simulink model "E3_QHW"  (R2025a)
settings: Solver=ode4  StartTime=0.0  StopTime=15  FixedStep=0.002  RelTol=1e-3  EnableMultiTasking=on
undefined symbols (not defined in the file): alpha_meas, g, HIL, Jp_cm, kt, l, mode, mp, mr, nis, p, qc_get_step_size, r, ref, Rm, seq, TET, theta_meas, tmodel, twall, Vm, xhat
libraries: quarc_library x7, simulink x6
settings Model: SimulationMode=external  ExtModeTrigDuration=10000  Creator=sebas  LastModifiedBy=sebas
settings SolverCC: AlgebraicLoopSolver=TrustRegion  PositivePriorityOrder=on
settings DataIOCC: ReturnWorkspaceOutputs=off
settings DebuggingCC: UnconnectedInputMsg=warning  UnconnectedOutputMsg=warning  UnconnectedLineMsg=warning  ArithmeticOperatorsInVariantConditions=warning
settings ModelReferenceCC: EnableRefExpFcnMdlSchedulingChecks=on
settings SFSimCC: SimUseLocalCustomCode=off  CustomCodeUndefinedFunction=UseInterfaceOnly
settings RTWCC: SystemTargetFile=quarc_win64.tlc  TemplateMakefile=quarc_default_tmf  RTWUseLocalCustomCode=off  Toolchain=QUARC win64 | nmake (64-bit Windows)  BuildConfiguration=Faster Runs  GPUComputeCapability=3.5  Description=QUARC Win64 Target Using Toolchain
settings CodeAppCC: StateflowObjectComments=on
settings STFCustomTargetCC: SystemTargetFile=quarc_win64.tlc  TargetLangStandard=C99 (ISO)  MultiwordLength=2048.0  DynamicStringBufferSize=256.0  ConcurrentExecutionCompliant=on  UseToolchainInfoCompliant=on
settings GRTTargetCC: ExtMode=on  ExtModeMexFile=quarc_comm  ParMdlRefBuildCompliant=off  CompOptLevelCompliant=off  CombineOutputUpdateFcns=off  MatFileLogging=off  CPPClassGenCompliant=off  GRTInterface=on
settings ConfigComp: CovMetricSettings=dswe

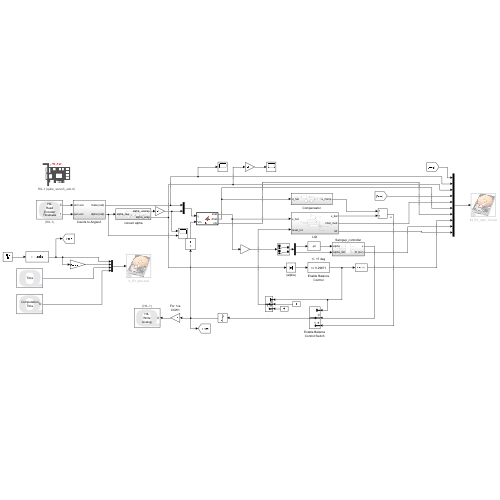
[thumbnail: Simulink's stored preview of the top-level diagram]
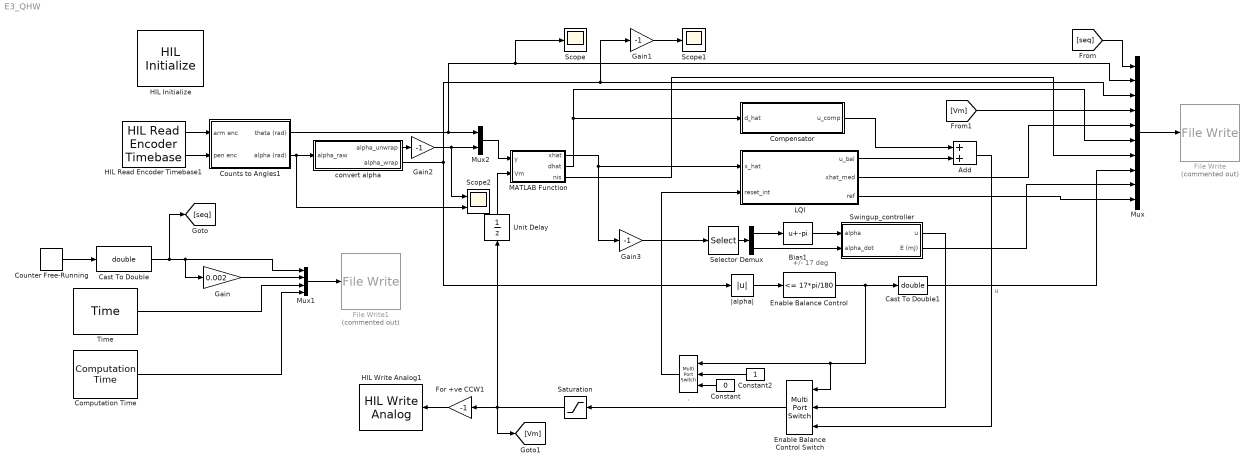
== system E3_QHW ==
  note: +/- 17 deg
  . : MultiPortSwitch  DataPortOrder=Zero-based contiguous  Inputs=2  zeroidx=on  SaturateOnIntegerOverflow=off  InputSameDT=off
  Add : Sum
  Bias1 : Bias  Bias=-pi  SaturateOnIntegerOverflow=off
  Cast To Double : DataTypeConversion  OutDataTypeStr=double  SaturateOnIntegerOverflow=off  RndMeth=Floor
  Cast To Double1 : DataTypeConversion  OutDataTypeStr=double  SaturateOnIntegerOverflow=off  RndMeth=Floor
  Compensator : Subsystem
  Computation Time : quarc_library/Sources/Time/Computation Time  sample_time=qc_get_step_size  use_model=on  use_cpu_time=off
  Constant : Constant  Value=0
  Constant2 : Constant
  Counter Free-Running : simulink/Sources/Counter Free-Running  NumBits=16  tsamp=0.002
  Counts to Angles1 : Subsystem
  Demux : Demux  Outputs=2
  Enable Balance Control : simulink/Logic and Bit Operations/Compare To Constant  relop=<=  const=17*pi/180  OutDataTypeStr=boolean  ZeroCross=off
  Enable Balance Control Switch : MultiPortSwitch  DataPortOrder=Zero-based contiguous  Inputs=2  zeroidx=on  SaturateOnIntegerOverflow=off  InputSameDT=off
  File Write : quarc_library/Sinks/To Target/File Write  Commented=on  source=Specify via dialog (do not evaluate)  file_name=fid_E3_qhw_10.mat  variable_name=seq,theta_meas,alpha_meas,Vm,xhat.dhat,nis,mode,E,ref  decimation=1  sample_time=0.002  file_format=MAT-file v.4  options=No header or footer  append=off  encoding=Default  bitrate=0
      settings: AttributesFormatString=%<file_name>  SourceProductName=QUARC Targets
  File Write1 : quarc_library/Sinks/To Target/File Write  Commented=on  source=Specify via dialog (do not evaluate)  file_name=rt_E3_qhw.mat  variable_name=seq,tmodel,twall,TET  decimation=1  sample_time=0.002  file_format=MAT-file v.4  options=No header or footer  append=off  encoding=Default  bitrate=0
      settings: AttributesFormatString=%<file_name>  SourceProductName=QUARC Targets
  For +ve CCW1 : Gain  Gain=-1
  Gain : Gain  Gain=0.002
  Gain1 : Gain  Gain=-1
  Gain2 : Gain  Gain=-1
  Gain3 : Gain  Gain=-1
  HIL Initialize : quarc_library/Data Acquisition/Generic/Configuration/HIL Initialize  object_name=HIL-1  board_type=qube_servo3_usb  board_number=0  board_options=deadband_compensation=0.3;pwm_en=0;enc0_velocity=3.0;enc1_velocity=3.0;min_diode_compensation=0.3;max_diode_compensation=1.5  exclusive=off  active=on  hardware_clocks=[0]  clock_modes=[]  initial_clock_frequencies=[]  set_clock_params_at_start=off  set_clock_params_at_switch_in=off  set_clock_frequencies_at_start=off  set_clock_frequencies_at_switch_in=off  analog_input_channels=[0]  analog_input_configurations=[]  analog_input_maximums=3  analog_input_minimums=-3  set_analog_input_params_at_start=off  set_analog_input_params_at_switch_in=off  analog_output_channels=[0]  analog_output_maximums=15  analog_output_minimums=-15  initial_analog_outputs=[0]  final_analog_outputs=[0]  watchdog_analog_outputs=0  set_analog_output_params_at_start=off  set_analog_output_params_at_switch_in=off  set_analog_outputs_at_start=on  set_analog_outputs_at_switch_in=off  set_analog_outputs_at_terminate=on  set_analog_outputs_at_switch_out=off  set_analog_outputs_on_watchdog=on  digital_input_channels=[]  digital_output_channels=[0]  digital_output_configuration=[]  initial_digital_outputs=[1]  final_digital_outputs=[0]  watchdog_digital_outputs=[0]  set_digital_output_params_at_start=off  set_digital_output_params_at_switch_in=off  set_digital_outputs_at_start=on  set_digital_outputs_at_switch_in=off  set_digital_outputs_at_terminate=on  set_digital_outputs_at_switch_out=off  set_digital_outputs_on_watchdog=on  encoder_channels=[0:1]  quadrature=[4]  encoder_filter_frequency=[]  initial_encoder_counts=[0]  set_encoder_params_at_start=off  set_encoder_params_at_switch_in=off  set_encoder_counts_at_start=on  set_encoder_counts_at_switch_in=off  pwm_channels=[]  pwm_modes=[0]  pwm_frequency=23195  pwm_configuration=[1]  pwm_alignment=[0]  pwm_polarity=[1]  pwm_leading_deadband=[0]  pwm_trailing_deadband=[0]  initial_pwm_outputs=[0]  final_pwm_outputs=[0]  watchdog_pwm_outputs=[]  set_pwm_params_at_start=off  set_pwm_params_at_switch_in=off  set_pwm_outputs_at_start=off  set_pwm_outputs_at_switch_in=off  set_pwm_outputs_at_terminate=off  set_pwm_outputs_at_switch_out=off  set_pwm_outputs_on_watchdog=off  other_output_channels=[11000:11002]  initial_other_outputs=[0 1 0]  final_other_outputs=[1 0 0]  watchdog_other_outputs=[0 0 1]  set_other_outputs_at_start=on  set_other_outputs_at_switch_in=off  set_other_outputs_at_terminate=on  set_other_outputs_at_switch_out=off  set_other_outputs_on_watchdog=on
  HIL Read Encoder Timebase1 : quarc_library/Data Acquisition/Generic/Timebases/HIL Read Encoder Timebase  object_name=HIL-1  clock=0  channels=[0:1]  active=on  vector_output=off  data_type_mode=Inherit via back propagation  data_type=double  overflow_mode=Error on overflow  samples_in_buffer=max(ceil(1/qc_get_step_size), 1)
  HIL Write Analog1 : quarc_library/Data Acquisition/Generic/Immediate I//O/HIL Write Analog  object_name=HIL-1  channels=0  sample_time=-1  active=off  vector_input=off
  LQI : Subsystem
  MATLAB Function : MATLAB Function  TreatAsAtomicUnit=on
  Mux : Mux  Inputs=10
  Mux1 : Mux
  Mux2 : Mux  Inputs=2
  Saturation : Saturate  UpperLimit=10  LowerLimit=-10
  Scope : Scope
      settings: ActiveDisplayYMinimum=-0.97599527629223914  ActiveDisplayYMaximum=1.5128885520522135
  Scope1 : Scope
      settings: ActiveDisplayYMinimum=-3.9235393602144986  ActiveDisplayYMaximum=3.9266073217902697
  Scope2 : Scope  NumInputPorts=2
      settings: ActiveDisplayYMinimum=-3.5165986422515694  ActiveDisplayYMaximum=6.5027597221689657  DataLoggingVariableName=ScopeData2
  Selector : Selector  InputPortWidth=4  IndexOptions=Index vector (dialog)  Indices=[2 4]  OutputSizes=1
  Swingup_controller : Subsystem
  Time : quarc_library/Sources/Time/Time  time_source=Wall clock  sample_time=qc_get_step_size
  Unit Delay : UnitDelay  SampleTime=-1  HasFrameUpgradeWarning=on
  convert alpha : Subsystem
  |alpha| : Abs  SaturateOnIntegerOverflow=off
  wires:
  Counter Free-Running/1 -> Cast To Double/1
  Gain/1 -> Mux1/2
  Time/1 -> Mux1/3
  Computation Time/1 -> Mux1/4
  Mux1/1 -> File Write1/1
  Cast To Double/1 -> [seq], Mux1/1, Gain/1
  Counts to Angles1/1(theta (rad)) -> Scope/1, Mux/2, Mux2/1
  Gain2/1 -> Scope2/1, Mux2/2
  Demux/1 -> Bias1/1
  Counts to Angles1/2(alpha (rad)) -> Scope2/2, convert alpha/1(alpha_raw)
  MATLAB Function/1(xhat) -> LQI/1(x_hat), Gain3/1
  HIL Read Encoder Timebase1/2 -> Counts to Angles1/2(pen enc)
  Unit Delay/1 -> MATLAB Function/2(Vm)
  Gain3/1 -> Selector/1
  ./1 -> LQI/2(reset_int)
  Selector/1 -> Demux/1
  Enable Balance Control/1 -> Enable Balance Control Switch/1, ./1, Cast To Double1/1
  Compensator/1(u_comp) -> Add/1
  Demux/2 -> Swingup_controller/2(alpha_dot)
  Mux2/1 -> MATLAB Function/1(y)
  For +ve CCW1/1 -> HIL Write Analog1/1
  Enable Balance Control Switch/1 -> Saturation/1
  Saturation/1 -> [Vm], Unit Delay/1, For +ve CCW1/1
  |alpha|/1 -> Enable Balance Control/1
  convert alpha/2(alpha_wrap) -> |alpha|/1, Gain1/1, Mux/3
  convert alpha/1(alpha_unwrap) -> Gain2/1
  Add/1 -> Enable Balance Control Switch/3  "u"
  MATLAB Function/2(dhat) -> Compensator/1(d_hat), Mux/6
  Bias1/1 -> Swingup_controller/1(alpha)
  LQI/1(u_bal) -> Add/2
  Constant2/1 -> ./2
  Swingup_controller/1(u) -> Enable Balance Control Switch/2
  HIL Read Encoder Timebase1/1 -> Counts to Angles1/1(arm enc)
  Constant/1 -> ./3
  [seq] -> Mux/1
  [Vm] -> Mux/4
  LQI/2(xhat_med) -> Mux/5
  MATLAB Function/3(nis) -> Mux/7
  Cast To Double1/1 -> Mux/8
  LQI/3(ref) -> Mux/10
  Swingup_controller/2(E (mJ)) -> Mux/9
  Mux/1 -> File Write/1
  Gain1/1 -> Scope1/1

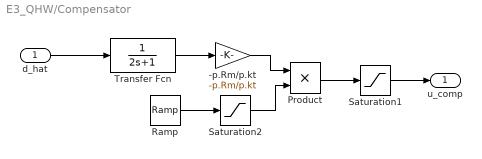
== system E3_QHW/Compensator ==
  d_hat : Inport
  -p.Rm/p.kt : Gain  Gain=-p.Rm/p.kt
  Product : Product
  Ramp : simulink/Sources/Ramp  slope=0.5  start=0  InitialOutput=0
  Saturation1 : Saturate  UpperLimit=2  LowerLimit=-2
  Saturation2 : Saturate  UpperLimit=1  LowerLimit=0
  Transfer Fcn : TransferFcn  Denominator=[2 1]
  u_comp : Outport
  wires:
  Saturation1/1 -> u_comp/1
  Transfer Fcn/1 -> -p.Rm/p.kt/1
  -p.Rm/p.kt/1 -> Product/1
  Saturation2/1 -> Product/2
  Ramp/1 -> Saturation2/1
  d_hat/1 -> Transfer Fcn/1
  Product/1 -> Saturation1/1

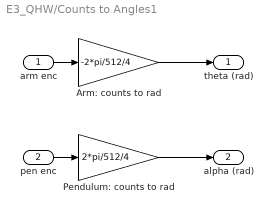
== system E3_QHW/Counts to Angles1 ==
  arm enc : Inport
  pen enc : Inport  Port=2
  Arm: counts to rad : Gain  Gain=-2*pi/512/4
  Pendulum: counts to rad : Gain  Gain=2*pi/512/4
  theta (rad) : Outport  VectorParamsAs1DForOutWhenUnconnected=off
  alpha (rad) : Outport  Port=2  VectorParamsAs1DForOutWhenUnconnected=off
  wires:
  pen enc/1 -> Pendulum: counts to rad/1
  arm enc/1 -> Arm: counts to rad/1
  Arm: counts to rad/1 -> theta (rad)/1
  Pendulum: counts to rad/1 -> alpha (rad)/1

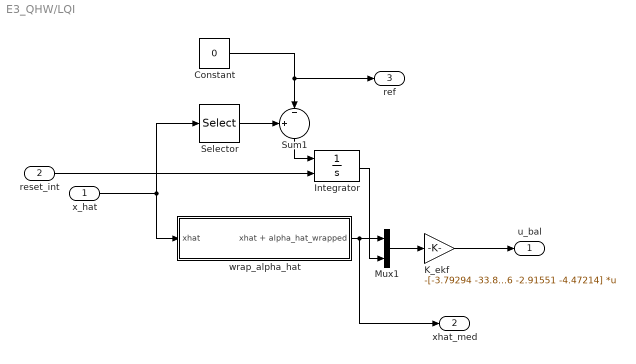
== system E3_QHW/LQI ==
  x_hat : Inport
  reset_int : Inport  Port=2
  Constant : Constant  Value=0
  Integrator : Integrator  ExternalReset=level hold  LimitOutput=on  UpperSaturationLimit=2  LowerSaturationLimit=-2
  K_ekf : Gain  Gain=-[-3.79294 -33.8988 -1.48036 -2.91551 -4.47214]  Multiplication=Matrix(K*u)
  Mux1 : Mux  Inputs=2
  Selector : Selector  InputPortWidth=4  IndexOptions=Index vector (dialog)  Indices=[1]  OutputSizes=1
  Sum1 : Sum  Inputs=+|-||
  wrap_alpha_hat : Subsystem
  u_bal : Outport
  xhat_med : Outport  Port=2
  ref : Outport  Port=3
  wires:
  Integrator/1 -> Mux1/2
  Mux1/1 -> K_ekf/1
  Constant/1 -> ref/1, Sum1/2
  Sum1/1 -> Integrator/1
  Selector/1 -> Sum1/1
  K_ekf/1 -> u_bal/1
  reset_int/1 -> Integrator/2
  x_hat/1 -> wrap_alpha_hat/1(xhat), Selector/1
  wrap_alpha_hat/1(xhat + alpha_hat_wrapped) -> xhat_med/1, Mux1/1

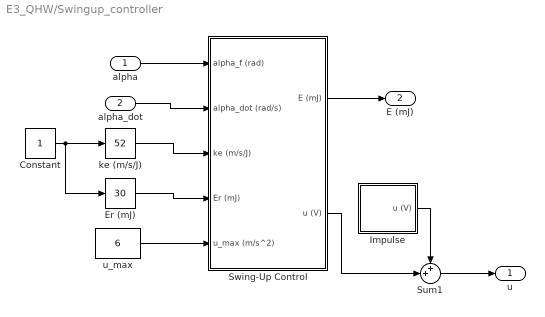
== system E3_QHW/Swingup_controller ==
  alpha : Inport
  alpha_dot : Inport  Port=2
  Constant : Constant
  Er (mJ) : simulink/Math Operations/Slider Gain  gain=30  low=0  high=100
  Impulse : Subsystem
  Sum1 : Sum  Inputs=++|
  Swing-Up Control : Subsystem
  ke (m/s/J) : simulink/Math Operations/Slider Gain  gain=52  low=0  high=100
  u_max : Constant  Value=6
  u : Outport
  E (mJ) : Outport  Port=2
  wires:
  alpha/1 -> Swing-Up Control/1(alpha_f (rad))
  Sum1/1 -> u/1
  u_max/1 -> Swing-Up Control/5(u_max (m/s^2))
  Impulse/1(u (V)) -> Sum1/1
  Swing-Up Control/1(E (mJ)) -> E (mJ)/1
  Swing-Up Control/2(u (V)) -> Sum1/2
  ke (m/s/J)/1 -> Swing-Up Control/3(ke (m/s/J))
  Constant/1 -> Er (mJ)/1, ke (m/s/J)/1
  Er (mJ)/1 -> Swing-Up Control/4(Er (mJ))
  alpha_dot/1 -> Swing-Up Control/2(alpha_dot (rad/s))

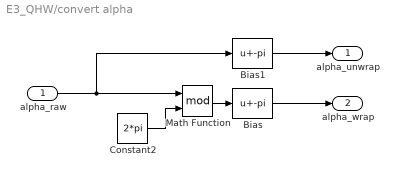
== system E3_QHW/convert alpha ==
  alpha_raw : Inport
  Bias : Bias  Bias=-pi  SaturateOnIntegerOverflow=off
  Bias1 : Bias  Bias=-pi  SaturateOnIntegerOverflow=off
  Constant2 : Constant  Value=2*pi
  Math Function : Math  Operator=mod  SignedPower=on
  alpha_unwrap : Outport
  alpha_wrap : Outport  Port=2
  wires:
  Math Function/1 -> Bias/1
  Bias/1 -> alpha_wrap/1
  Constant2/1 -> Math Function/2
  alpha_raw/1 -> Bias1/1, Math Function/1
  Bias1/1 -> alpha_unwrap/1

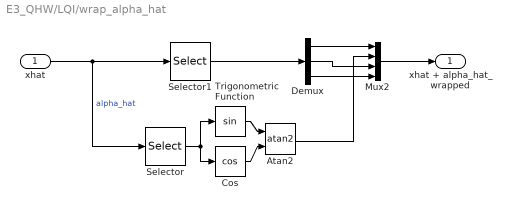
== system E3_QHW/LQI/wrap_alpha_hat ==
  xhat : Inport
  Atan2 : Trigonometry  Operator=atan2
  Cos : Trigonometry  Operator=cos
  Demux : Demux  Outputs=3
  Mux2 : Mux
  Selector : Selector  InputPortWidth=4  IndexOptions=Index vector (dialog)  Indices=[2]  OutputSizes=1
  Selector1 : Selector  InputPortWidth=4  IndexOptions=Index vector (dialog)  Indices=[1 3 4]  OutputSizes=1
  Trigonometric Function : Trigonometry
  xhat + alpha_hat_wrapped : Outport
  wires:
  Selector/1 -> Cos/1, Trigonometric Function/1
  Mux2/1 -> xhat + alpha_hat_wrapped/1
  Cos/1 -> Atan2/2
  xhat/1 -> Selector/1, Selector1/1  "alpha_hat"
  Trigonometric Function/1 -> Atan2/1
  Demux/2 -> Mux2/3
  Selector1/1 -> Demux/1
  Demux/1 -> Mux2/1
  Demux/3 -> Mux2/4
  Atan2/1 -> Mux2/2

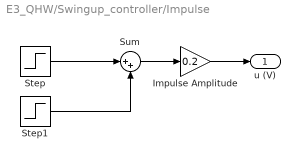
== system E3_QHW/Swingup_controller/Impulse ==
  Impulse Amplitude : Gain  Gain=0.2
  Step : Step  SampleTime=0
  Step1 : Step  Time=1.1  After=-1  SampleTime=0
  Sum : Sum  Inputs=|++
  u (V) : Outport  VectorParamsAs1DForOutWhenUnconnected=off
  wires:
  Impulse Amplitude/1 -> u (V)/1
  Sum/1 -> Impulse Amplitude/1
  Step/1 -> Sum/1
  Step1/1 -> Sum/2

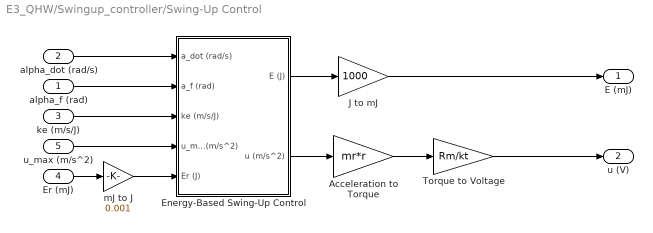
== system E3_QHW/Swingup_controller/Swing-Up Control ==
  alpha_f (rad) : Inport
  alpha_dot (rad/s) : Inport  Port=2
  ke (m/s/J) : Inport  Port=3
  Er (mJ) : Inport  Port=4
  u_max (m/s^2) : Inport  Port=5
  Acceleration to Torque : Gain  Gain=mr*r
  Energy-Based Swing-Up Control : Subsystem
  J to mJ : Gain  Gain=1000
  Torque to Voltage : Gain  Gain=Rm/kt
  mJ to J : Gain  Gain=0.001
  E (mJ) : Outport  VectorParamsAs1DForOutWhenUnconnected=off
  u (V) : Outport  Port=2  VectorParamsAs1DForOutWhenUnconnected=off
  wires:
  mJ to J/1 -> Energy-Based Swing-Up Control/5(Er (J))
  alpha_dot (rad/s)/1 -> Energy-Based Swing-Up Control/1(a_dot (rad/s))
  Torque to Voltage/1 -> u (V)/1
  J to mJ/1 -> E (mJ)/1
  Er (mJ)/1 -> mJ to J/1
  Acceleration to Torque/1 -> Torque to Voltage/1
  u_max (m/s^2)/1 -> Energy-Based Swing-Up Control/4(u_max (m/s^2))
  ke (m/s/J)/1 -> Energy-Based Swing-Up Control/3(ke (m/s/J))
  alpha_f (rad)/1 -> Energy-Based Swing-Up Control/2(a_f (rad))
  Energy-Based Swing-Up Control/1(E (J)) -> J to mJ/1
  Energy-Based Swing-Up Control/2(u (m/s^2)) -> Acceleration to Torque/1

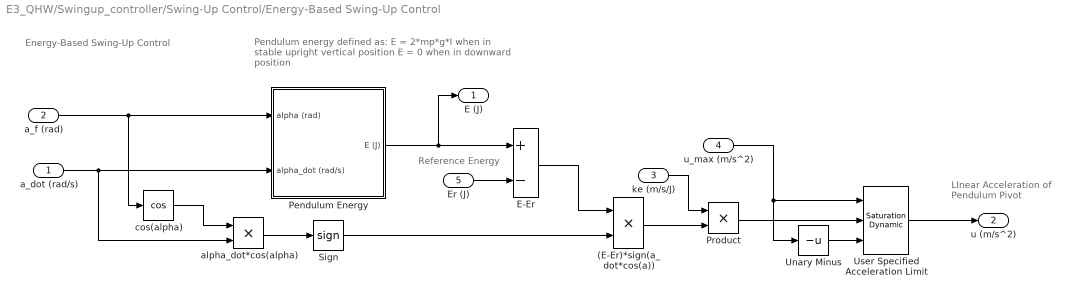
== system E3_QHW/Swingup_controller/Swing-Up Control/Energy-Based Swing-Up Control ==
  note: Pendulum energy defined as:
      | E = 2*mp*g*l when in stable upright vertical position
      | E = 0 when in downward position
  note: Reference Energy
  note: LInear Acceleration of
      | Pendulum Pivot
  note: Energy-Based Swing-Up Control
  a_dot (rad/s) : Inport
  a_f (rad) : Inport  Port=2
  ke (m/s/J) : Inport  Port=3
  u_max (m/s^2) : Inport  Port=4
  Er (J) : Inport  Port=5
  (E-Er)*sign(a_dot*cos(a)) : Product  RndMeth=Zero
  E-Er : Sum  Inputs=+-
  Pendulum Energy : Subsystem
  Product : Product  RndMeth=Zero
  Sign : Signum
  Unary Minus : UnaryMinus
  User Specified Acceleration Limit : simulink/Discontinuities/Saturation Dynamic  OutMin=[]  OutMax=[]  OutDataTypeStr=Inherit: Same as second input  OutDataType=fixdt(1, 16)  OutScaling=2^-10  DoSatur=off
  alpha_dot*cos(alpha) : Product  RndMeth=Zero
  cos(alpha) : Trigonometry  Operator=cos
  E (J) : Outport  VectorParamsAs1DForOutWhenUnconnected=off
  u (m/s^2) : Outport  Port=2  VectorParamsAs1DForOutWhenUnconnected=off
  wires:
  User Specified Acceleration Limit/1 -> u (m/s^2)/1
  Unary Minus/1 -> User Specified Acceleration Limit/3
  u_max (m/s^2)/1 -> Unary Minus/1, User Specified Acceleration Limit/1
  Product/1 -> User Specified Acceleration Limit/2
  ke (m/s/J)/1 -> Product/1
  Er (J)/1 -> E-Er/2
  (E-Er)*sign(a_dot*cos(a))/1 -> Product/2
  a_dot (rad/s)/1 -> Pendulum Energy/2(alpha_dot (rad/s)), alpha_dot*cos(alpha)/2
  Pendulum Energy/1(E (J)) -> E-Er/1, E (J)/1
  E-Er/1 -> (E-Er)*sign(a_dot*cos(a))/1
  cos(alpha)/1 -> alpha_dot*cos(alpha)/1
  alpha_dot*cos(alpha)/1 -> Sign/1
  Sign/1 -> (E-Er)*sign(a_dot*cos(a))/2
  a_f (rad)/1 -> cos(alpha)/1, Pendulum Energy/1(alpha (rad))

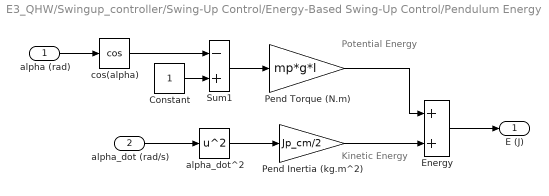
== system E3_QHW/Swingup_controller/Swing-Up Control/Energy-Based Swing-Up Control/Pendulum Energy ==
  note: Potential Energy
  note: Kinetic Energy
  alpha (rad) : Inport
  alpha_dot (rad/s) : Inport  Port=2
  Constant : Constant
  Energy : Sum  SaturateOnIntegerOverflow=on
  Pend Inertia (kg.m^2) : Gain  Gain=Jp_cm/2
  Pend Torque (N.m) : Gain  Gain=mp*g*l
  Sum1 : Sum  Inputs=-+  SaturateOnIntegerOverflow=on
  alpha_dot^2 : Math  Operator=square  SignedPower=on
  cos(alpha) : Trigonometry  Operator=cos
  E (J) : Outport  VectorParamsAs1DForOutWhenUnconnected=off
  wires:
  cos(alpha)/1 -> Sum1/1
  Energy/1 -> E (J)/1
  alpha_dot (rad/s)/1 -> alpha_dot^2/1
  alpha (rad)/1 -> cos(alpha)/1
  Pend Torque (N.m)/1 -> Energy/1
  alpha_dot^2/1 -> Pend Inertia (kg.m^2)/1
  Pend Inertia (kg.m^2)/1 -> Energy/2
  Constant/1 -> Sum1/2
  Sum1/1 -> Pend Torque (N.m)/1

== matlab function E3_QHW/MATLAB Function ==
  settings: updateMethod=DISCRETE  sampleTime=0.002
  data: y input; xhat output; Vm input; dhat output; nis output
function [xhat, dhat,nis] = fcn(y, Vm)
   [xhat, dhat,nis] = ekf_step(y, Vm);
end
